simulink model "Assignment2Simulation"  (R2017b)
settings: Solver=FixedStepAuto  StartTime=0.0  StopTime=6000  FixedStep=2  RelTol=1e-2
values from neighbouring files (symbols this model uses):
  A = 1    [Assignment2Script.m]
  Cd = 2.7    [Assignment2Script.m]
  H = 50e3    (= 50000)    [Assignment2Script.m]
  h0 = 200e3    (= 200000)    [Assignment2Script.m]
  m = 600    [Assignment2Script.m]
  mu = 3.98694e14    (= 398694000000000)    [Assignment2Script.m]
  Ra = 6387135    [Assignment2Script.m]
  rho0 = 3e-10    [Assignment2Script.m]
  vx0 = 0    [Assignment2Script.m]
  vy0 = 7.616e3    (= 7616)    [Assignment2Script.m]
  x0 = Ra+500e3    (= 6887135)    [Assignment2Script.m]
  y0 = 0    [Assignment2Script.m]
settings Model: Creator=Niels  LastModifiedBy=Niels
settings DataIOCC: SaveOutput=off  SignalLogging=off  DSMLogging=off

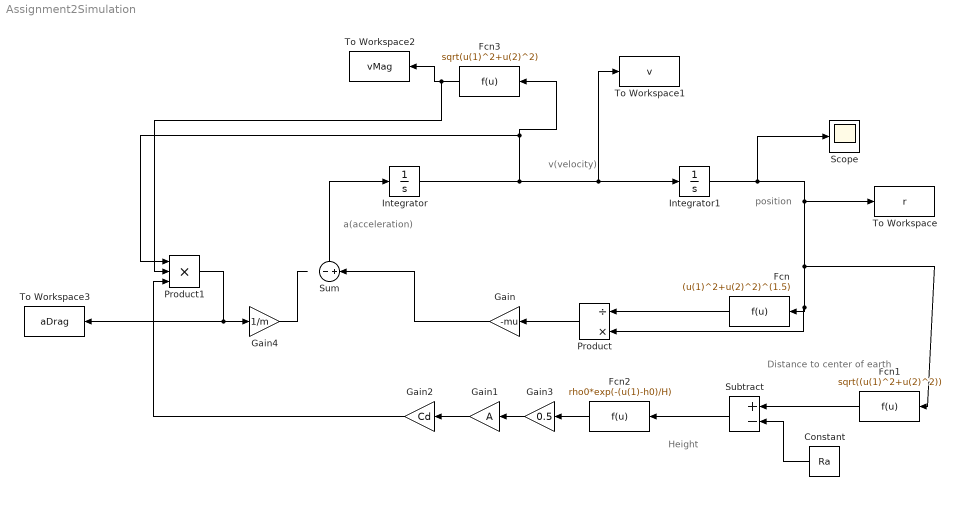
== system Assignment2Simulation ==
  note: Height
  note: Distance to center of earth
  note: position
  note: v(velocity)
  note: a(acceleration)
  Constant : Constant  Value=Ra
  Fcn : Fcn  Expr=(u(1)^2+u(2)^2)^(1.5)
  Fcn1 : Fcn  Expr=sqrt((u(1)^2+u(2)^2))
  Fcn2 : Fcn  Expr=rho0*exp(-(u(1)-h0)/H)
  Fcn3 : Fcn  Expr=sqrt(u(1)^2+u(2)^2)
  Gain : Gain  Gain=-mu
  Gain1 : Gain  Gain=A
  Gain2 : Gain  Gain=Cd
  Gain3 : Gain  Gain=0.5
  Gain4 : Gain  Gain=1/m
  Integrator : Integrator  InitialCondition=[vx0,vy0]
  Integrator1 : Integrator  InitialCondition=[x0,y0]
  Product : Product  Inputs=/*
  Product1 : Product  Inputs=3
  Scope : Scope
  Subtract : Sum  Inputs=+-
  Sum : Sum  Inputs=-+
  To Workspace : ToWorkspace  VariableName=r  SampleTime=-1
      settings: Save2DSignal=2-D array (concatenate along first dimension)
  To Workspace1 : ToWorkspace  VariableName=v  SampleTime=-1
      settings: Save2DSignal=2-D array (concatenate along first dimension)
  To Workspace2 : ToWorkspace  VariableName=vMag  SaveFormat=Timeseries  SampleTime=-1
  To Workspace3 : ToWorkspace  VariableName=aDrag  SampleTime=-1
      settings: Save2DSignal=2-D array (concatenate along first dimension)
  wires:
  Integrator/1 -> Product1/1, Fcn3/1, To Workspace1/1, Integrator1/1
  Integrator1/1 -> Scope/1, To Workspace/1, Fcn1/1, Product/2, Fcn/1
  Fcn/1 -> Product/1
  Product/1 -> Gain/1
  Gain/1 -> Sum/2
  Fcn1/1 -> Subtract/1
  Constant/1 -> Subtract/2
  Subtract/1 -> Fcn2/1
  Gain3/1 -> Gain1/1
  Fcn2/1 -> Gain3/1
  Gain1/1 -> Gain2/1
  Sum/1 -> Integrator/1
  Fcn3/1 -> Product1/2, To Workspace2/1
  Product1/1 -> Gain4/1, To Workspace3/1
  Gain2/1 -> Product1/3
  Gain4/1 -> ?
